simulink model "simple_switch"  (R2023b)
settings: Solver=VariableStepAuto  StartTime=0.0  StopTime=10.0  RelTol=1e-3
settings Model: Creator=39216  LastModifiedBy=39216

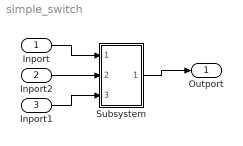
== system simple_switch ==
  Inport : Inport
  Inport2 : Inport  Port=2
  Inport1 : Inport  Port=3
  Subsystem : Subsystem
  Outport : Outport
  wires:
  Subsystem/1(Outport) -> Outport/1
  Inport/1 -> Subsystem/1(Inport)
  Inport1/1 -> Subsystem/3(Inport1)
  Inport2/1 -> Subsystem/2(Inport2)

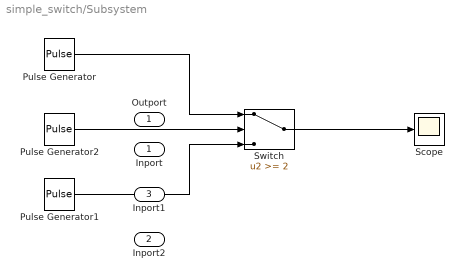
== system simple_switch/Subsystem ==
  Inport : Inport
  Inport2 : Inport  Port=2
  Inport1 : Inport  Port=3
  Pulse Generator : DiscretePulseGenerator  PulseType=Time based  Period=10  PulseWidth=50
  Pulse Generator1 : DiscretePulseGenerator  PulseType=Time based  Amplitude=2  Period=10  PulseWidth=50  PhaseDelay=5
  Pulse Generator2 : DiscretePulseGenerator  PulseType=Time based  Period=10  PulseWidth=5
  Scope : Scope
  Switch : Switch  Threshold=2  SaturateOnIntegerOverflow=off  InputSameDT=off
  Outport : Outport
  wires:
  Pulse Generator/1 -> Switch/1
  Switch/1 -> Scope/1
  Pulse Generator1/1 -> Switch/3
  Pulse Generator2/1 -> Switch/2
